simulink model "neighobserver"  (R2021a)
settings: Solver=VariableStepAuto  StartTime=0.0  StopTime=50  MaxStep=0.005
values from neighbouring files (symbols this model uses):
  A = adj    [ceren_function.m]    (also in deneme.m = [A_1 ;A_2; A_3;A_4; A_5;A_6])
  B = [B_1; B_2; B_3; B_4; B_5; B_6]    [deneme.m]
  B_dist = 2*[0; 0.0717; 0; -0.7374; 0; 1.9776]    [deneme.m]
  c = 1    [init_graph.m]
  C1 = [0.0717 0 -0.7374 0 1.9776 0]    [deneme.m]
  C2 = [0.0699 0 -0.5958 0 1.2029 0]    [deneme.m]
  C3 = [0.0665 0 -0.4444 0 0.4020 0]    [deneme.m]
  C4 = [0.0630 0 -0.2977 0 -0.3216 0]    [deneme.m]
  D = [0 0 0 0]    [deneme.m]
  F1 = -F1'    [init_graph.m]
  F2 = -F2'    [init_graph.m]
  F3 = -F3'    [init_graph.m]
  F4 = -F4'    [init_graph.m]
  K = kron(A, B)    [kronecker.m]
  w1 = 2*pi* 0.2745    (= 1.72473436682)    [deneme.m]
  w2 = 2*pi* 2.9446    (= 18.5014674555)    [deneme.m]
settings Model: Creator=umut  LastModifiedBy=umut

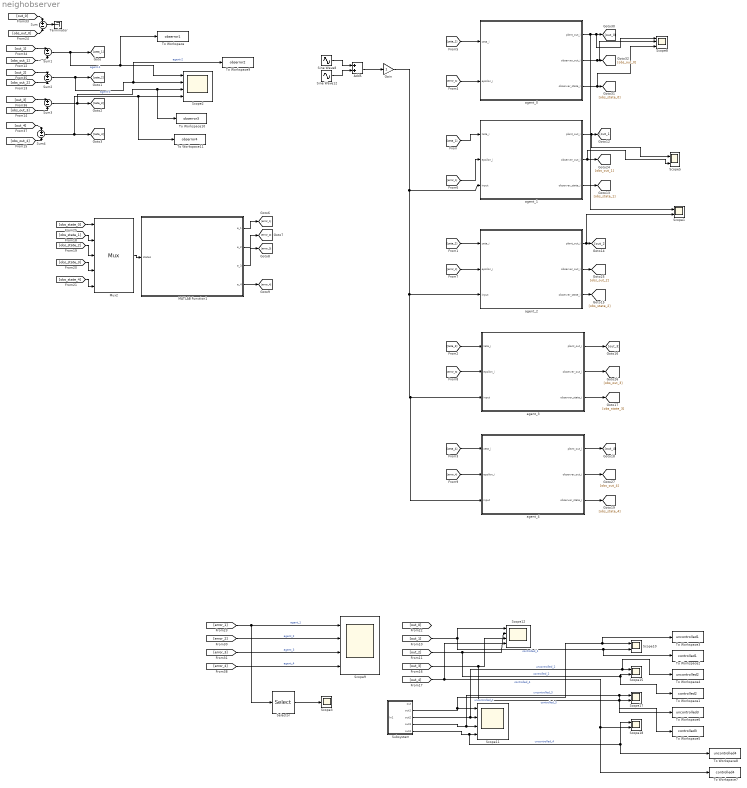
== system neighobserver ==
  Add5 : Sum
  Gain : Gain
  MATLAB Function1 : MATLAB Function  TreatAsAtomicUnit=on
  Mux2 : Mux  Inputs=5
  Scope{1,5,10,15,17..18} (6 alike) : Scope  NumInputPorts=2
  Scope{2,9,11..12} (4 alike) : Scope  NumInputPorts=4
  Scope3 : Scope
  Scope8 : Scope  NumInputPorts=6
  Selector : Selector  InputPortWidth=6  IndexOptions=Starting index (dialog)  Indices=4  OutputSizes=1
  Sine Wave12 : Sin  Amplitude=0.5  Frequency=w2  SampleTime=0
  Sine Wave8 : Sin  Amplitude=0.5  Frequency=w1  SampleTime=0
  Subsystem : Subsystem
  Sum{,1..4} (5 alike) : Sum  Inputs=+|-
  Terminator : Terminator
  To Workspace : ToWorkspace  VariableName=obserror1  SampleTime=-1
      settings: Save2DSignal=2-D array (concatenate along first dimension)
  To Workspace1 : ToWorkspace  VariableName=controlled2  SampleTime=-1
      settings: Save2DSignal=2-D array (concatenate along first dimension)
  To Workspace10 : ToWorkspace  VariableName=obserror3  SampleTime=-1
      settings: Save2DSignal=2-D array (concatenate along first dimension)
  To Workspace11 : ToWorkspace  VariableName=obserror4  SampleTime=-1
      settings: Save2DSignal=2-D array (concatenate along first dimension)
  To Workspace2 : ToWorkspace  VariableName=controlled1  SampleTime=-1
      settings: Save2DSignal=2-D array (concatenate along first dimension)
  To Workspace3 : ToWorkspace  VariableName=uncontrolled1  SampleTime=-1
      settings: Save2DSignal=2-D array (concatenate along first dimension)
  To Workspace4 : ToWorkspace  VariableName=uncontrolled2  SampleTime=-1
      settings: Save2DSignal=2-D array (concatenate along first dimension)
  To Workspace5 : ToWorkspace  VariableName=controlled3  SampleTime=-1
      settings: Save2DSignal=2-D array (concatenate along first dimension)
  To Workspace6 : ToWorkspace  VariableName=uncontrolled3  SampleTime=-1
      settings: Save2DSignal=2-D array (concatenate along first dimension)
  To Workspace7 : ToWorkspace  VariableName=controlled4  SampleTime=-1
      settings: Save2DSignal=2-D array (concatenate along first dimension)
  To Workspace8 : ToWorkspace  VariableName=uncontrolled4  SampleTime=-1
      settings: Save2DSignal=2-D array (concatenate along first dimension)
  To Workspace9 : ToWorkspace  VariableName=obserror2  SampleTime=-1
      settings: Save2DSignal=2-D array (concatenate along first dimension)
  agent_0 : Subsystem
  agent_1 : Subsystem
  agent_2 : Subsystem
  agent_3 : Subsystem
  agent_4 : Subsystem
  wires:
  [obs_out_1] -> Sum1/2
  MATLAB Function1/2(e_2) -> [error_2]
  [out_3] -> Sum3/1
  [out_2] -> Sum2/1
  [obs_out_2] -> Sum2/2
  [obs_state_3] -> Mux2/4
  [obs_state_2] -> Mux2/3
  [out_4] -> Sum4/1
  [obs_state_1] -> Mux2/2
  MATLAB Function1/4(e_4) -> [error_4]
  MATLAB Function1/3(e_3) -> [error_3]
  Mux2/1 -> MATLAB Function1/1(states)
  MATLAB Function1/1(e_1) -> [error_1]
  [out_0] -> Sum/1
  [obs_out_0] -> Sum/2
  [out_1] -> Sum1/1
  [obs_state_0] -> Mux2/1
  [obs_out_4] -> Sum4/2
  [obs_out_3] -> Sum3/2
  [obs_state_4] -> Mux2/5
  Sum4/1 -> To Workspace11/1, Scope2/4, [zeta_4]
  Sum/1 -> Terminator/1
  agent_4/3(observer_state_i) -> [obs_state_4]
  agent_1/3(observer_state_i) -> [obs_state_1]
  agent_4/2(observer_out_i) -> [obs_out_4]
  [zeta_4] -> agent_4/1(zeta_i)
  agent_3/1(plant_out_i) -> [out_3]
  [zeta_1] -> agent_0/1(zeta_i)
  [zeta_2] -> agent_2/1(zeta_i)
  agent_1/1(plant_out_i) -> Scope5/1, [out_1]
  [zeta_3] -> agent_3/1(zeta_i)
  [error_1] -> agent_1/2(epsilon_i)
  [error_2] -> agent_2/2(epsilon_i)
  [error_1] -> agent_0/2(epsilon_i)
  agent_4/1(plant_out_i) -> [out_4]
  agent_3/3(observer_state_i) -> [obs_state_3]
  agent_3/2(observer_out_i) -> [obs_out_3]
  agent_2/1(plant_out_i) -> Scope1/2, [out_2]
  [zeta_1] -> agent_1/1(zeta_i)
  agent_2/3(observer_state_i) -> [obs_state_2]
  agent_0/2(observer_out_i) -> Scope8/3, [obs_out_0]
  agent_2/2(observer_out_i) -> [obs_out_2]
  agent_0/3(observer_state_i) -> Scope8/6, [obs_state_0]
  Gain/1 -> agent_4/3(input), agent_3/3(input), agent_2/3(input), agent_1/3(input)
  agent_0/1(plant_out_i) -> Scope1/1, Scope8/1, [out_0]
  [error_3] -> agent_3/2(epsilon_i)
  [error_4] -> agent_4/2(epsilon_i)
  agent_1/2(observer_out_i) -> Scope5/2, [obs_out_1]
  Add5/1 -> Gain/1
  Sine Wave8/1 -> Add5/1
  Sine Wave12/1 -> Add5/2
  [out_1] -> Scope12/1, To Workspace2/1, Scope10/2  "controlled_1"
  [out_3] -> To Workspace5/1, Scope17/2, Scope12/3  "controlled_3"
  Subsystem/3(out2) -> To Workspace4/1, Scope15/1, Scope11/2  "uncontrolled_2"
  [error_4] -> Scope9/4  "agent_4"
  [out_4] -> To Workspace7/1, Scope18/2, Scope12/4  "controlled_4"
  [out_2] -> To Workspace1/1, Scope15/2, Scope12/2  "controlled_2"
  Selector/1 -> Scope3/1
  Subsystem/4(out3) -> To Workspace6/1, Scope17/1, Scope11/3  "uncontrolled_3"
  Subsystem/5(out4) -> Scope18/1, To Workspace8/1, Scope11/4  "uncontrolled_4"
  Subsystem/2(out1) -> To Workspace3/1, Scope10/1, Scope11/1  "uncontrolled_1"
  [error_3] -> Scope9/3  "agent_3"
  [error_1] -> Selector/1, Scope9/1  "agent_1"
  [error_2] -> Scope9/2  "agent_2"
  Sum3/1 -> To Workspace10/1, Scope2/3, [zeta_3]  "agent-3"
  Sum1/1 -> To Workspace/1, Scope2/1, [zeta_1]  "agent-1"
  Sum2/1 -> To Workspace9/1, Scope2/2, [zeta_2]  "agent-2"

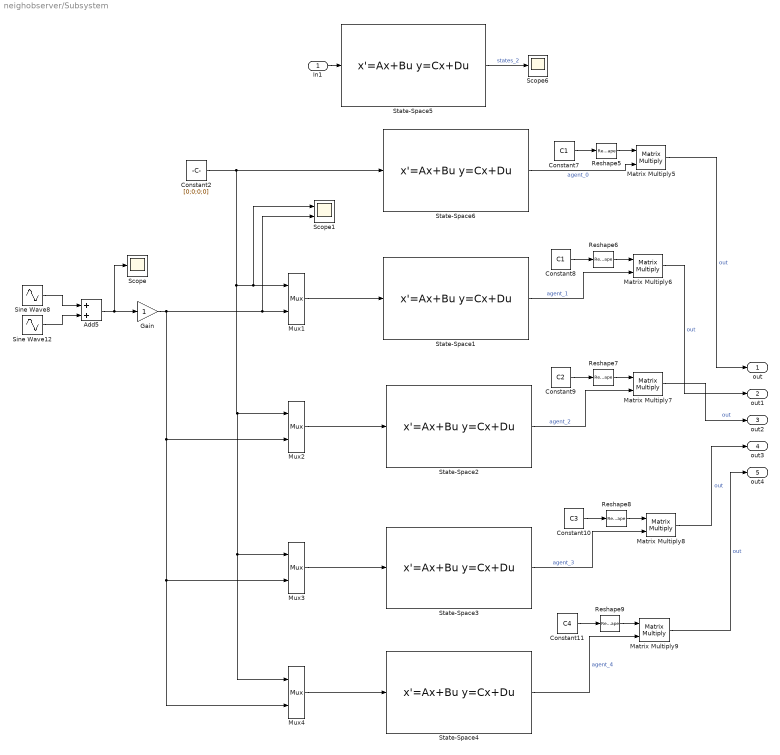
== system neighobserver/Subsystem ==
  In1 : Inport
  Add5 : Sum
  Constant10 : Constant  Value=C3
  Constant11 : Constant  Value=C4
  Constant2 : Constant  Value=[0;0;0;0]
  Constant7 : Constant  Value=C1
  Constant8 : Constant  Value=C1
  Constant9 : Constant  Value=C2
  Gain : Gain
  Matrix Multiply{5..9} (5 alike) : Product  Multiplication=Matrix(*)
  Mux{1..4} (4 alike) : Mux  Inputs=2
  Reshape{5..9} (5 alike) : Reshape  OutputDimensionality=Customize  OutputDimensions=[1,6]
  Scope : Scope
  Scope1 : Scope  NumInputPorts=2
  Scope6 : Scope
  Sine Wave12 : Sin  Amplitude=0.5  Frequency=w2  SampleTime=0
  Sine Wave8 : Sin  Amplitude=0.5  Frequency=w1  SampleTime=0
  State-Space1 : StateSpace  A=A  B=[B B_dist]  C=eye(6)  D=[D 0;D 0;D 0;D 0;D 0;D 0]  InitialCondition=[0.1;0.2;0.3;0.4;0.5;0.6]
  State-Space2 : StateSpace  A=A  B=[B B_dist]  C=eye(6)  D=[D 0;D 0;D 0;D 0;D 0;D 0]  InitialCondition=[0.6;0.5;0.4;0.3;0.2;0.1]
  State-Space3 : StateSpace  A=A  B=[B B_dist]  C=eye(6)  D=[D 0;D 0;D 0;D 0;D 0;D 0]  InitialCondition=[0.6;0.3;0.1;0.4;0;0.8]
  State-Space4 : StateSpace  A=A  B=[B B_dist]  C=eye(6)  D=[D 0;D 0;D 0;D 0;D 0;D 0]  InitialCondition=[0.3;0.1;0.7;0.2;0.8;0.4]
  State-Space5 : StateSpace  A=A  B=B  C=eye(6)  D=[D;D;D;D;D;D]  InitialCondition=[1,2,3,4,5,6]
  State-Space6 : StateSpace  A=A  B=B  C=eye(6)  D=[D;D;D;D;D;D]  InitialCondition=[0.1;0.2;0.3;0.4;0.5;0.6]
  out : Outport
  out1 : Outport  Port=2
  out2 : Outport  Port=3
  out3 : Outport  Port=4
  out4 : Outport  Port=5
  wires:
  State-Space2/1 -> Matrix Multiply7/2  "agent_2"
  Constant11/1 -> Reshape9/1
  Constant7/1 -> Reshape5/1
  State-Space3/1 -> Matrix Multiply8/2  "agent_3"
  Matrix Multiply8/1 -> out3/1  "out"
  Matrix Multiply9/1 -> out4/1  "out"
  Reshape8/1 -> Matrix Multiply8/1
  Constant9/1 -> Reshape7/1
  In1/1 -> State-Space5/1
  Reshape5/1 -> Matrix Multiply5/1
  State-Space4/1 -> Matrix Multiply9/2  "agent_4"
  State-Space1/1 -> Matrix Multiply6/2  "agent_1"
  Matrix Multiply7/1 -> out2/1  "out"
  Reshape6/1 -> Matrix Multiply6/1
  Constant8/1 -> Reshape6/1
  State-Space5/1 -> Scope6/1  "states_2"
  Matrix Multiply6/1 -> out1/1  "out"
  Constant10/1 -> Reshape8/1
  Reshape9/1 -> Matrix Multiply9/1
  Matrix Multiply5/1 -> out/1  "out"
  Reshape7/1 -> Matrix Multiply7/1
  State-Space6/1 -> Matrix Multiply5/2  "agent_0"
  Mux4/1 -> State-Space4/1
  Mux3/1 -> State-Space3/1
  Sine Wave12/1 -> Add5/2
  Sine Wave8/1 -> Add5/1
  Mux1/1 -> State-Space1/1
  Mux2/1 -> State-Space2/1
  Add5/1 -> Gain/1, Scope/1
  Constant2/1 -> Mux4/1, Mux3/1, Mux2/1, Scope1/1, Mux1/1, State-Space6/1
  Gain/1 -> Mux4/2, Mux3/2, Mux2/2, Scope1/2, Mux1/2

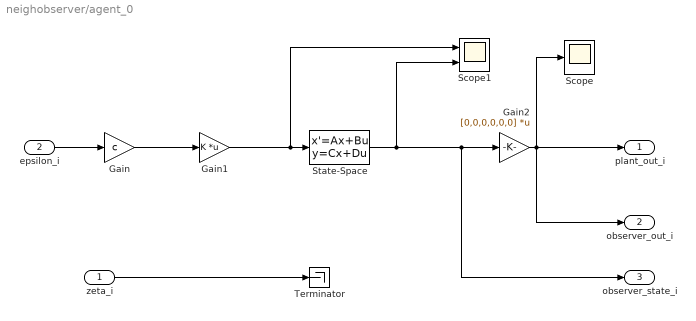
== system neighobserver/agent_0 ==
  zeta_i : Inport
  epsilon_i : Inport  Port=2
  Gain : Gain  Gain=c
  Gain1 : Gain  Gain=K  Multiplication=Matrix(K*u)
  Gain2 : Gain  Gain=[0,0,0,0,0,0]  Multiplication=Matrix(K*u)
  Scope : Scope
  Scope1 : Scope  NumInputPorts=2
  State-Space : StateSpace  A=A  B=B  C=zeros(6)  D=zeros(6,4)  InitialCondition=[0.1;0.2;0.3;0.4;0.5;0.6]
  Terminator : Terminator
  plant_out_i : Outport
  observer_out_i : Outport  Port=2
  observer_state_i : Outport  Port=3
  wires:
  epsilon_i/1 -> Gain/1
  zeta_i/1 -> Terminator/1
  State-Space/1 -> Scope1/2, Gain2/1, observer_state_i/1
  Gain/1 -> Gain1/1
  Gain2/1 -> Scope/1, plant_out_i/1, observer_out_i/1
  Gain1/1 -> Scope1/1, State-Space/1

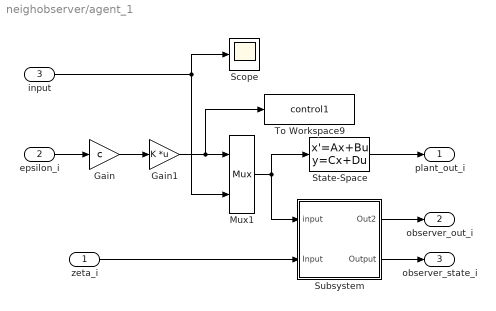
== system neighobserver/agent_1 ==
  zeta_i : Inport
  epsilon_i : Inport  Port=2
  input : Inport  Port=3
  Gain : Gain  Gain=c
  Gain1 : Gain  Gain=K  Multiplication=Matrix(K*u)
  Mux1 : Mux  Inputs=2
  Scope : Scope
  State-Space : StateSpace  A=A  B=[B B_dist]  C=C1  D=[D 0]  InitialCondition=[0.1;0.2;0.3;0.4;0.5;0.6]
  Subsystem : Subsystem
  To Workspace9 : ToWorkspace  VariableName=control1  SampleTime=-1
      settings: Save2DSignal=2-D array (concatenate along first dimension)
  plant_out_i : Outport
  observer_out_i : Outport  Port=2
  observer_state_i : Outport  Port=3
  wires:
  epsilon_i/1 -> Gain/1
  State-Space/1 -> plant_out_i/1
  Subsystem/1(Out2) -> observer_out_i/1
  Subsystem/2(Output) -> observer_state_i/1
  zeta_i/1 -> Subsystem/2(Input)
  Gain/1 -> Gain1/1
  Mux1/1 -> State-Space/1, Subsystem/1(input)
  Gain1/1 -> To Workspace9/1, Mux1/1
  input/1 -> Scope/1, Mux1/2

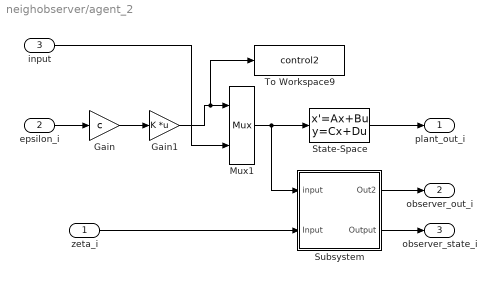
== system neighobserver/agent_2 ==
  zeta_i : Inport
  epsilon_i : Inport  Port=2
  input : Inport  Port=3
  Gain : Gain  Gain=c
  Gain1 : Gain  Gain=K  Multiplication=Matrix(K*u)
  Mux1 : Mux  Inputs=2
  State-Space : StateSpace  A=A  B=[B B_dist]  C=C2  D=[D 0]  InitialCondition=[0.6;0.5;0.4;0.3;0.2;0.1]
  Subsystem : Subsystem
  To Workspace9 : ToWorkspace  VariableName=control2  SampleTime=-1
      settings: Save2DSignal=2-D array (concatenate along first dimension)
  plant_out_i : Outport
  observer_out_i : Outport  Port=2
  observer_state_i : Outport  Port=3
  wires:
  epsilon_i/1 -> Gain/1
  State-Space/1 -> plant_out_i/1
  Subsystem/1(Out2) -> observer_out_i/1
  Subsystem/2(Output) -> observer_state_i/1
  zeta_i/1 -> Subsystem/2(Input)
  Gain/1 -> Gain1/1
  Mux1/1 -> Subsystem/1(input), State-Space/1
  Gain1/1 -> To Workspace9/1, Mux1/1
  input/1 -> Mux1/2

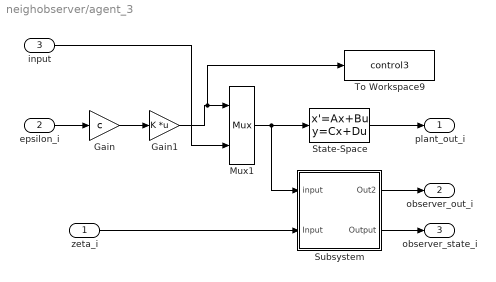
== system neighobserver/agent_3 ==
  zeta_i : Inport
  epsilon_i : Inport  Port=2
  input : Inport  Port=3
  Gain : Gain  Gain=c
  Gain1 : Gain  Gain=K  Multiplication=Matrix(K*u)
  Mux1 : Mux  Inputs=2
  State-Space : StateSpace  A=A  B=[B B_dist]  C=C3  D=[D 0]  InitialCondition=[0.6;0.3;0.1;0.4;0;0.8]
  Subsystem : Subsystem
  To Workspace9 : ToWorkspace  VariableName=control3  SampleTime=-1
      settings: Save2DSignal=2-D array (concatenate along first dimension)
  plant_out_i : Outport
  observer_out_i : Outport  Port=2
  observer_state_i : Outport  Port=3
  wires:
  epsilon_i/1 -> Gain/1
  State-Space/1 -> plant_out_i/1
  Subsystem/1(Out2) -> observer_out_i/1
  Subsystem/2(Output) -> observer_state_i/1
  zeta_i/1 -> Subsystem/2(Input)
  Gain/1 -> Gain1/1
  Mux1/1 -> Subsystem/1(input), State-Space/1
  Gain1/1 -> To Workspace9/1, Mux1/1
  input/1 -> Mux1/2

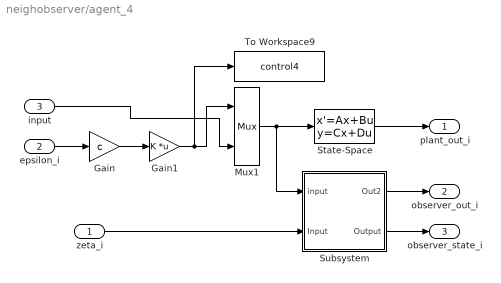
== system neighobserver/agent_4 ==
  zeta_i : Inport
  epsilon_i : Inport  Port=2
  input : Inport  Port=3
  Gain : Gain  Gain=c
  Gain1 : Gain  Gain=K  Multiplication=Matrix(K*u)
  Mux1 : Mux  Inputs=2
  State-Space : StateSpace  A=A  B=[B B_dist]  C=C4  D=[D 0]  InitialCondition=[0.3;0.1;0.7;0.2;0.8;0.4]
  Subsystem : Subsystem
  To Workspace9 : ToWorkspace  VariableName=control4  SampleTime=-1
      settings: Save2DSignal=2-D array (concatenate along first dimension)
  plant_out_i : Outport
  observer_out_i : Outport  Port=2
  observer_state_i : Outport  Port=3
  wires:
  epsilon_i/1 -> Gain/1
  State-Space/1 -> plant_out_i/1
  Subsystem/1(Out2) -> observer_out_i/1
  Subsystem/2(Output) -> observer_state_i/1
  zeta_i/1 -> Subsystem/2(Input)
  Gain/1 -> Gain1/1
  Mux1/1 -> Subsystem/1(input), State-Space/1
  Gain1/1 -> To Workspace9/1, Mux1/1
  input/1 -> Mux1/2

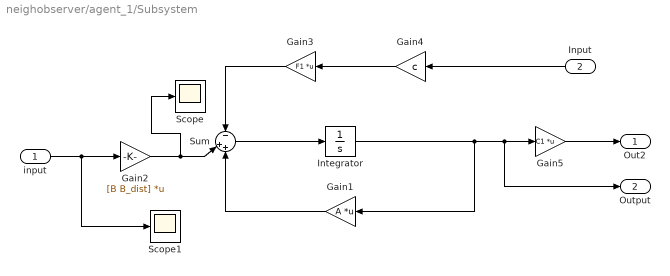
== system neighobserver/agent_1/Subsystem ==
  input : Inport
  Input : Inport  Port=2
  Gain1 : Gain  Gain=A  Multiplication=Matrix(K*u)
  Gain2 : Gain  Gain=[B B_dist]  Multiplication=Matrix(K*u)
  Gain3 : Gain  Gain=F1  Multiplication=Matrix(K*u)
  Gain4 : Gain  Gain=c
  Gain5 : Gain  Gain=C1  Multiplication=Matrix(K*u)
  Integrator : Integrator
  Scope : Scope
  Scope1 : Scope
  Sum : Sum  Inputs=-|++
  Out2 : Outport
  Output : Outport  Port=2
  wires:
  Gain3/1 -> Sum/1
  Gain2/1 -> Scope/1, Sum/2
  Gain1/1 -> Sum/3
  Sum/1 -> Integrator/1
  Gain5/1 -> Out2/1
  Input/1 -> Gain4/1
  Gain4/1 -> Gain3/1
  Integrator/1 -> Output/1, Gain5/1, Gain1/1
  input/1 -> Scope1/1, Gain2/1

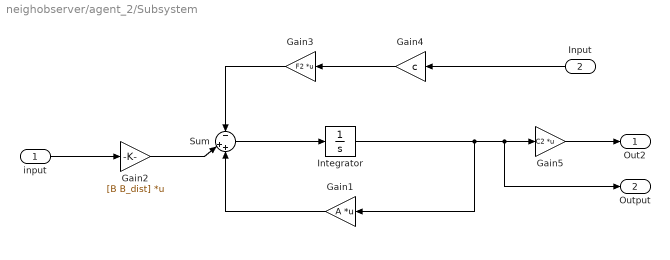
== system neighobserver/agent_2/Subsystem ==
  input : Inport
  Input : Inport  Port=2
  Gain1 : Gain  Gain=A  Multiplication=Matrix(K*u)
  Gain2 : Gain  Gain=[B B_dist]  Multiplication=Matrix(K*u)
  Gain3 : Gain  Gain=F2  Multiplication=Matrix(K*u)
  Gain4 : Gain  Gain=c
  Gain5 : Gain  Gain=C2  Multiplication=Matrix(K*u)
  Integrator : Integrator
  Sum : Sum  Inputs=-|++
  Out2 : Outport
  Output : Outport  Port=2
  wires:
  Gain3/1 -> Sum/1
  Gain2/1 -> Sum/2
  input/1 -> Gain2/1
  Gain1/1 -> Sum/3
  Sum/1 -> Integrator/1
  Gain5/1 -> Out2/1
  Input/1 -> Gain4/1
  Gain4/1 -> Gain3/1
  Integrator/1 -> Output/1, Gain5/1, Gain1/1

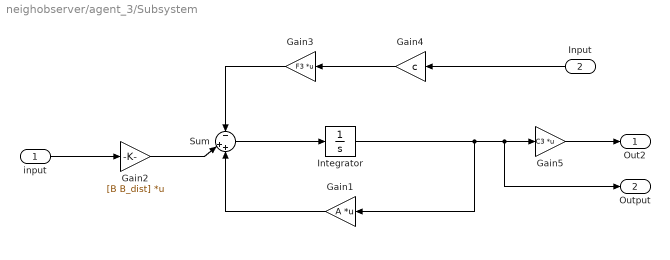
== system neighobserver/agent_3/Subsystem ==
  input : Inport
  Input : Inport  Port=2
  Gain1 : Gain  Gain=A  Multiplication=Matrix(K*u)
  Gain2 : Gain  Gain=[B B_dist]  Multiplication=Matrix(K*u)
  Gain3 : Gain  Gain=F3  Multiplication=Matrix(K*u)
  Gain4 : Gain  Gain=c
  Gain5 : Gain  Gain=C3  Multiplication=Matrix(K*u)
  Integrator : Integrator
  Sum : Sum  Inputs=-|++
  Out2 : Outport
  Output : Outport  Port=2
  wires:
  Gain3/1 -> Sum/1
  Gain2/1 -> Sum/2
  input/1 -> Gain2/1
  Gain1/1 -> Sum/3
  Sum/1 -> Integrator/1
  Gain5/1 -> Out2/1
  Input/1 -> Gain4/1
  Gain4/1 -> Gain3/1
  Integrator/1 -> Output/1, Gain5/1, Gain1/1

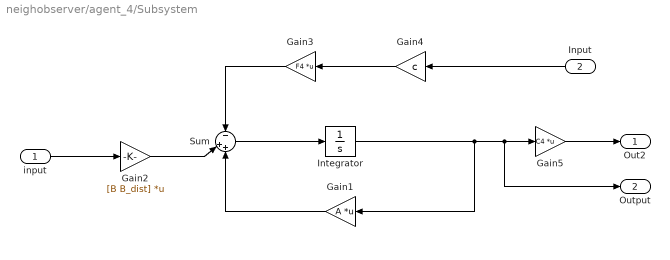
== system neighobserver/agent_4/Subsystem ==
  input : Inport
  Input : Inport  Port=2
  Gain1 : Gain  Gain=A  Multiplication=Matrix(K*u)
  Gain2 : Gain  Gain=[B B_dist]  Multiplication=Matrix(K*u)
  Gain3 : Gain  Gain=F4  Multiplication=Matrix(K*u)
  Gain4 : Gain  Gain=c
  Gain5 : Gain  Gain=C4  Multiplication=Matrix(K*u)
  Integrator : Integrator
  Sum : Sum  Inputs=-|++
  Out2 : Outport
  Output : Outport  Port=2
  wires:
  Gain3/1 -> Sum/1
  Gain2/1 -> Sum/2
  input/1 -> Gain2/1
  Gain1/1 -> Sum/3
  Sum/1 -> Integrator/1
  Gain5/1 -> Out2/1
  Input/1 -> Gain4/1
  Gain4/1 -> Gain3/1
  Integrator/1 -> Output/1, Gain5/1, Gain1/1

== matlab function neighobserver/MATLAB Function1 ==
  data: states input; e_1 output size=[6 1]; e_2 output size=[6 1]; e_3 output size=[6 1]; e_4 output size=[6 1]
function [e_1, e_2, e_3, e_4]  = calculate_neighborhood_error(states)
    adj = [ 0	0	0	0
            1   0   1   0
            1   0   0   1
            1   1   0   0]
    
    pinnings = [1; 0; 0; 0];

    A = adj;
    G = pinnings;
    
    size_agents = 4;
    size_states = 6;
    
    error = zeros(size_states, size_agents);
    
    
    for i = 1 : size_agents
        error_temp = [0;0;0;0;0;0];
        for j = 1 : size_agents
            error_temp = error_temp + A(i, j) * (states((j)*6+1 : 6*(j+1)) - states((i)*6+1 : 6*(i+1)));
        end
        error_temp = error_temp + pinnings(i) * (states(1 : 6) - states((i)*6+1 : 6*(i+1)));
        error(:,i) = error_temp;
    end
    
    e_1 = error(:,1);
    e_2 = error(:,2);
    e_3 = error(:,3);
    e_4 = error(:,4);

end
